simulink model "ideal_Motor"  (R2018b)
settings: Solver=VariableStepAuto  StartTime=0.0  StopTime=10.0  RelTol=1e-3
undefined symbols (not defined in the file): Jm, Ld, Lq, Phia, Pn, Ra, taul, wrm2rpm
settings Model: Creator=81803  LastModifiedBy=81803

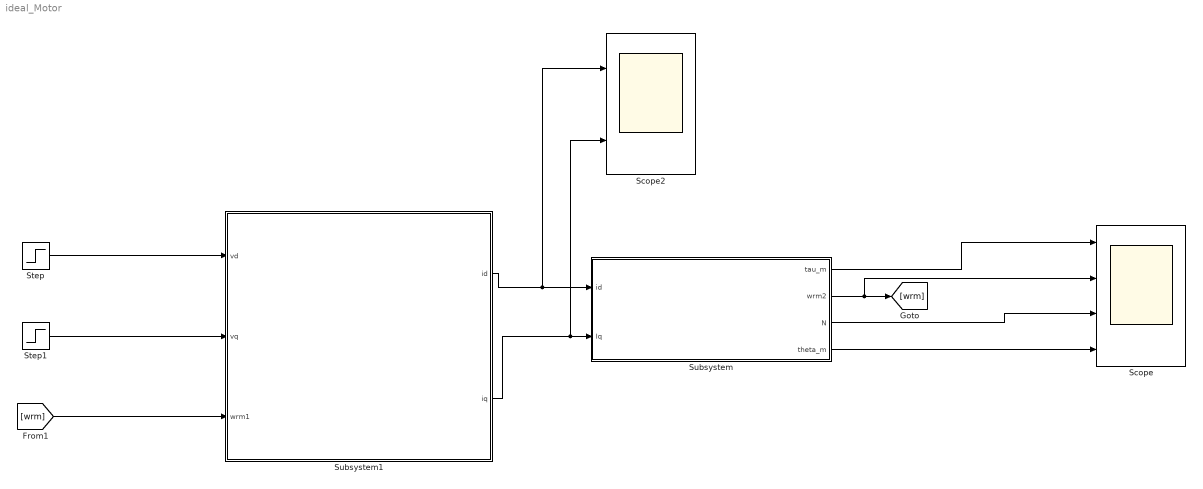
== system ideal_Motor ==
  Scope : Scope  NumInputPorts=4
  Scope2 : Scope  NumInputPorts=2
  Step : Step  After=0  SampleTime=0
  Step1 : Step  SampleTime=0
  Subsystem : Subsystem
  Subsystem1 : Subsystem
  wires:
  Subsystem/2(wrm2) -> [wrm], Scope/2
  Subsystem1/2(iq) -> Subsystem/2(Iq), Scope2/2
  [wrm] -> Subsystem1/3(wrm1)
  Subsystem1/1(id) -> Scope2/1, Subsystem/1(id)
  Subsystem/1(tau_m) -> Scope/1
  Subsystem/3(N) -> Scope/3
  Subsystem/4(theta_m) -> Scope/4
  Step/1 -> Subsystem1/1(vd)
  Step1/1 -> Subsystem1/2(vq)

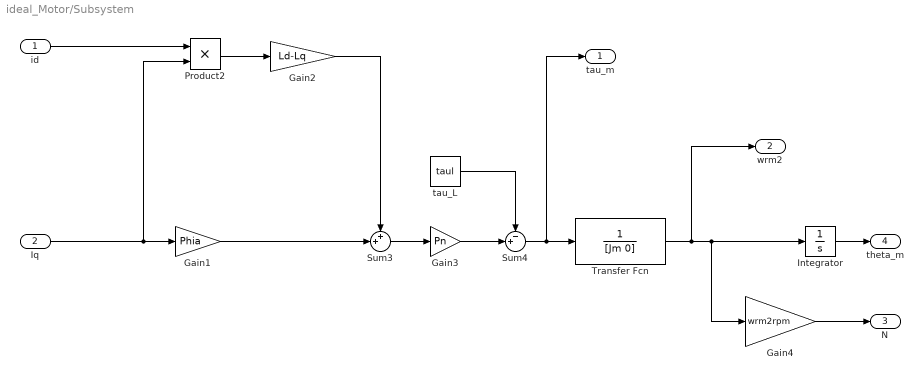
== system ideal_Motor/Subsystem ==
  id : Inport
  Iq : Inport  Port=2
  Gain1 : Gain  Gain=Phia
  Gain2 : Gain  Gain=Ld-Lq
  Gain3 : Gain  Gain=Pn
  Gain4 : Gain  Gain=wrm2rpm
  Integrator : Integrator
  Product2 : Product
  Sum3 : Sum  Inputs=++|
  Sum4 : Sum  Inputs=-+|
  Transfer Fcn : TransferFcn  Denominator=[Jm 0]
  tau_L : Constant  Value=taul
  tau_m : Outport
  wrm2 : Outport  Port=2
  N : Outport  Port=3
  theta_m : Outport  Port=4
  wires:
  Product2/1 -> Gain2/1
  Sum3/1 -> Gain3/1
  Gain2/1 -> Sum3/1
  Iq/1 -> Product2/2, Gain1/1
  id/1 -> Product2/1
  Gain1/1 -> Sum3/2
  Transfer Fcn/1 -> wrm2/1, Gain4/1, Integrator/1
  Sum4/1 -> tau_m/1, Transfer Fcn/1
  Gain3/1 -> Sum4/2
  tau_L/1 -> Sum4/1
  Integrator/1 -> theta_m/1
  Gain4/1 -> N/1

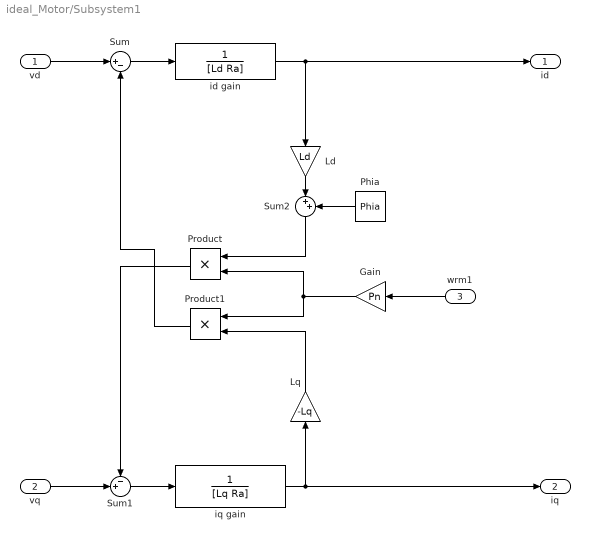
== system ideal_Motor/Subsystem1 ==
  vd : Inport
  vq : Inport  Port=2
  wrm1 : Inport  Port=3
  Gain : Gain  Gain=Pn
  Ld : Gain  Gain=Ld
  Lq : Gain  Gain=-Lq
  Phia : Constant  Value=Phia
  Product : Product
  Product1 : Product
  Sum : Sum  Inputs=|+-
  Sum1 : Sum  Inputs=-+|
  Sum2 : Sum  Inputs=|++
  id gain : TransferFcn  Denominator=[Ld Ra]
  iq gain : TransferFcn  Denominator=[Lq Ra]
  id : Outport
  iq : Outport  Port=2
  wires:
  Gain/1 -> Product1/1, Product/2
  Phia/1 -> Sum2/2
  Sum1/1 -> iq gain/1
  Product/1 -> Sum1/1
  Sum2/1 -> Product/1
  id gain/1 -> id/1, Ld/1
  Product1/1 -> Sum/2
  Lq/1 -> Product1/2
  iq gain/1 -> Lq/1, iq/1
  wrm1/1 -> Gain/1
  vd/1 -> Sum/1
  Ld/1 -> Sum2/1
  Sum/1 -> id gain/1
  vq/1 -> Sum1/2
